simulink model "SVPWM_simulink1"  (R2022a)
settings: Solver=ode23tb  StartTime=0.0  StopTime=0.1  MaxStep=0.00001  RelTol=1e-3  EnableMultiTasking=on
InitFcn:
  | Vdc=700;
libraries: spsSVPWMGenerator2LevelLib x1, spspowerguiLib x1
settings Model: Creator=Lei  LastModifiedBy=25313
settings SolverCC: AlgebraicLoopSolver=TrustRegion
settings DataIOCC: LimitDataPoints=on  SaveFormat=Array  ReturnWorkspaceOutputs=off
settings OptimizationCC: LifeSpan=inf
settings DebuggingCC: SolverPrmCheckMsg=warning  UnconnectedInputMsg=warning  UnconnectedOutputMsg=warning  UnconnectedLineMsg=warning  SFUnexpectedBacktrackingDiag=warning  SFNoUnconditionalDefaultTransitionDiag=warning  SFExecutionAtInitializationDiag=none  SFMachineParentedDataDiag=warning  ArithmeticOperatorsInVariantConditions=warning
settings HardwareCC: ProdBitPerPointer=32  ProdBitPerSizeT=32  ProdBitPerPtrDiffT=32  ProdLargestAtomicFloat=None  ProdIntDivRoundTo=Undefined  ProdEndianess=Unspecified  ProdWordSize=32  ProdHWDeviceType=32-bit Generic
settings ModelReferenceCC: PropagateSignalLabelsOutOfModel=off
settings SFSimCC: SimUseLocalCustomCode=off  CustomCodeUndefinedFunction=UseInterfaceOnly
settings RTWCC: RTWUseLocalCustomCode=off
settings CodeAppCC: StateflowObjectComments=on
settings GRTTargetCC: TargetLangStandard=C89/C90 (ANSI)
settings ConfigComp: CovMetricSettings=dw  CovSaveCumulativeToWorkspaceVar=on  CovSaveSingleToWorkspaceVar=on  CovExternalEMLEnable=off  CovSFcnEnable=off

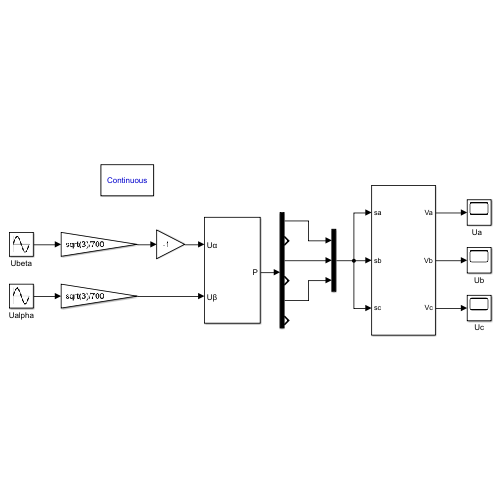
[thumbnail: Simulink's stored preview of the top-level diagram]
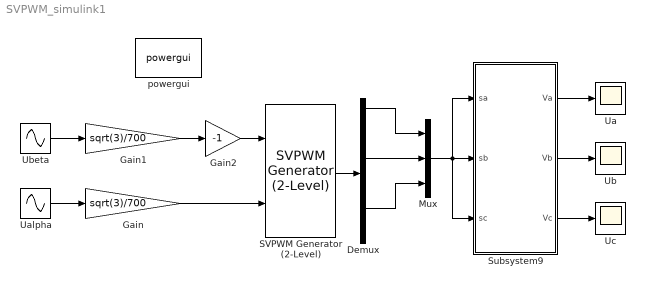
== system SVPWM_simulink1 ==
  Demux : Demux  Outputs=6
  Gain : Gain  Gain=sqrt(3)/700
  Gain1 : Gain  Gain=sqrt(3)/700
  Gain2 : Gain  Gain=-1
  Mux : Mux  Inputs=3
  SVPWM Generator (2-Level) : spsSVPWMGenerator2LevelLib/SVPWM Generator (2-Level)  InputType=alpha-beta components  SwitchingPattern=Pattern #1  Fc=5000  ParUref=[0.8 -30 50]  Ts=0
      settings: SourceProductBaseCode=PS
  Subsystem9 : Subsystem
  "Ua  " : Scope
  Ualpha : Sin  Amplitude=200  Frequency=100*pi  Phase=pi/2  SampleTime=0
  Ub : Scope
  Ubeta : Sin  Amplitude=200  Frequency=100*pi  SampleTime=0
  Uc : Scope
  powergui : spspowerguiLib/powergui  Priority=1  SimulationMode=Continuous  SampleTime=50e-6  frequency=60  Iterations=50  frequencyindice=60  Pbase=100e6  ErrMax=1e-4  UnitsV=kV  UnitsW=MW  buscounter=0  FunctionMessages=off  echomessages=off  EnableUseOfTLC=off  CurrentSourceSwitches=on  DisableSnubberDevices=off  DisableRonSwitches=off  DisableVfSwitches=off  DisplayEquations=off  AutomaticDiscreteSolvers=off  SolverType=Tustin/Backward Euler (TBE)  Interpol=off  ExternalGateDelay=off  methode=off  Ts=100  x0status=blocks  SPID=off  SwTol=0  HookPort=off  NonlinearTolerance=1e-4  nMaxIteration=100  ContinueOnMaxIteration=off  RestoreLinks=warning  ResistiveCurrentMeasurement=off  Frange=[0:2:500]  Ylog=off  Xlog=on  ShowGrid=off  save=off  variable=ZData  structure=Ua  ZoomFFT=off  StartTime=0.05  cycles=1  DisplayStyle=1  fundamental=50  FreqAxis=off  MaxFrequency=9000  frequencyindicesteady=1  RmsSteady=1  display=off
  wires:
  Ualpha/1 -> Gain/1
  Ubeta/1 -> Gain1/1
  Subsystem9/1(Va) -> "Ua  "/1
  Subsystem9/2(Vb) -> Ub/1
  Subsystem9/3(Vc) -> Uc/1
  SVPWM Generator (2-Level)/1 -> Demux/1
  Demux/1 -> Mux/1
  Demux/3 -> Mux/2
  Demux/5 -> Mux/3
  Mux/1 -> Subsystem9/1(sa), Subsystem9/3(sc), Subsystem9/2(sb)
  Gain1/1 -> Gain2/1
  Gain/1 -> SVPWM Generator (2-Level)/2
  Gain2/1 -> SVPWM Generator (2-Level)/1

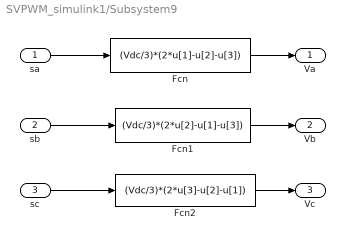
== system SVPWM_simulink1/Subsystem9 ==
  sa : Inport
  sb : Inport  Port=2
  sc : Inport  Port=3
  Fcn : Fcn  Expr=(Vdc/3)*(2*u[1]-u[2]-u[3])
  Fcn1 : Fcn  Expr=(Vdc/3)*(2*u[2]-u[1]-u[3])
  Fcn2 : Fcn  Expr=(Vdc/3)*(2*u[3]-u[2]-u[1])
  Va : Outport
  Vb : Outport  Port=2
  Vc : Outport  Port=3
  wires:
  Fcn/1 -> Va/1
  Fcn1/1 -> Vb/1
  Fcn2/1 -> Vc/1
  sa/1 -> Fcn/1
  sb/1 -> Fcn1/1
  sc/1 -> Fcn2/1
